simulink model "FLIGHT_Hexacopter_V2"  (R2025a)
settings: Solver=FixedStepDiscrete  StartTime=0.0  StopTime=inf  FixedStep=SampleTime_SAS  RelTol=1e-3  EnableMultiTasking=on
InitFcn:
  | Init_FLIGHT_Hexacopter
values from neighbouring files (symbols this model uses):
  d2r = pi/180    (= 0.0174532925199)    [Init_FLIGHT_Hexacopter.m]
  Kdrr = 0.004    [Init_FLIGHT_Hexacopter_fromNCMS.m]
  Kirr = 0.0    (= 0)    [Init_FLIGHT_Hexacopter_fromNCMS.m]
  Kpp = 3.3894    [Init_FLIGHT_Hexacopter_fromNCMS.m]
  Kpr = 3.3894    [Init_FLIGHT_Hexacopter_fromNCMS.m]
  Kprr = 0.1    [Init_FLIGHT_Hexacopter_fromNCMS.m]
  MAX_CONTROL_ANGLE_PITCH = 30*pi/180    (= 0.523598775598)    [Init_FLIGHT_Hexacopter.m]    (also in Init_FLIGHT_Hexacopter_fromNCMS.m = 0.349065850399)
  MAX_CONTROL_ANGLE_RATE_PITCH = 360*pi/180    (= 6.28318530718)    [Init_FLIGHT_Hexacopter.m]    (also in Init_FLIGHT_Hexacopter_fromNCMS.m)
  MAX_CONTROL_ANGLE_RATE_ROLL = 360*pi/180    (= 6.28318530718)    [Init_FLIGHT_Hexacopter.m]    (also in Init_FLIGHT_Hexacopter_fromNCMS.m)
  MAX_CONTROL_ANGLE_RATE_Y = 120*pi/180    (= 2.09439510239)    [Init_FLIGHT_Hexacopter.m]    (also in Init_FLIGHT_Hexacopter_fromNCMS.m)
  MAX_CONTROL_ANGLE_ROLL = 30*pi/180    (= 0.523598775598)    [Init_FLIGHT_Hexacopter.m]    (also in Init_FLIGHT_Hexacopter_fromNCMS.m = 0.349065850399)
  Nrr = 50    [Init_FLIGHT_Hexacopter_fromNCMS.m]
  PITCH_AUTHORITY = 1    [Init_FLIGHT_Hexacopter.m]
  ROLL_AUTHORITY = 1    [Init_FLIGHT_Hexacopter.m]
  SampleTime = 1/250    (= 0.004)    [Init_FLIGHT_Hexacopter.m]    (also in Init_FLIGHT_Hexacopter_fromNCMS.m = 0.01)
  SampleTime_SAS = 1/1000    (= 0.001)    [Init_FLIGHT_Hexacopter.m]
  YAW_AUTHORITY = 1    [Init_FLIGHT_Hexacopter.m]
undefined symbols (not defined in the file or in its folder): arguments, DiscIntNeverNeededParam, e_dot, event_sequence, fx, g1x, hx, id, integral_e, log_levels, MPC_Z_D, MPC_Z_I, MPC_Z_P, noutputs, omega, omega_dot, output, phi_cmd, phi_cmd_ddot, phi_cmd_dot, r, s, tau_roll, timestamp, w
libraries: px4Utilslib x65, simulink x21, px4uORBlib x12, slpidlib x9, cstblocks x5, simulink_extras x2, sharedtransform x1, px4Sensorslib x1, matrix_library x1, px4Peripheralslib x1
(part 1 of 3)
settings Model: ExtModeTrigDuration=10  Creator=sslee  LastModifiedBy=sslee
settings SolverCC: AlgebraicLoopSolver=TrustRegion  PositivePriorityOrder=on  MaxZcPerStep=1.0
settings OptimizationCC: EnhancedBackFolding=on  PassReuseOutputArgsAs=Individual arguments  ZeroExternalMemoryAtStartup=off  ZeroInternalMemoryAtStartup=off  MaxStackSize=64  OptimizeBlockOrder=speed  DifferentSizesBufferReuse=on  OptimizationCustomize=off  EfficientTunableParamExpr=on
settings DebuggingCC: ParameterTunabilityLossMsg=error  UnconnectedInputMsg=warning  UnconnectedOutputMsg=warning  UnconnectedLineMsg=warning  SymbolicDimsDataTypeCodeGenerationDiagnostic=none
settings HardwareCC: ProdBitPerPointer=32.0  ProdBitPerSizeT=32.0  ProdBitPerPtrDiffT=32.0  ProdLargestAtomicInteger=Long  ProdLargestAtomicFloat=Double  ProdWordSize=32.0  ProdLongLongMode=on  ProdHWDeviceType=ARM Compatible->ARM Cortex
settings ModelReferenceCC: EnableRefExpFcnMdlSchedulingChecks=on
settings SFSimCC: MATLABDynamicMemAlloc=off  SimTargetLang=C++  SimDLTargetLibrary=mkl-dnn
settings RTWCC: SystemTargetFile=ert.tlc  HardwareBoard=PX4 Pixhawk 6x  TLCOptions="-aInlineSetEventsForThisBaseRateFcn=TLC_FALSE -aSuppressMultiTaskScheduler=TLC_FALSE  -aRateBasedStepFcn=0"  TemplateMakefile=ert_default_tmf  GenerateReport=on  Toolchain=GNU Tools for PX4 Autopilots  IncludeHyperlinkInReport=on  LaunchReport=on  TargetLang=C++  GPUComputeCapability=3.5  DLArmComputeVersion=19.05  Description=Embedded Coder
settings CodeAppCC: ForceParamTrailComments=on  IgnoreCustomStorageClasses=off  OperatorAnnotations=on  SimulinkDataObjDesc=on  SFDataObjDesc=on  MATLABFcnDesc=on  InsertBlockDesc=on  BlockCommentType=BlockSIDComment  MATLABSourceComments=on
settings ERTTargetCC: ExtModeTransport=3.0  ExtModeStaticAllocSize=1024.0  InlinedParameterPlacement=Hierarchical  DynamicArrayContainerType=coder::array

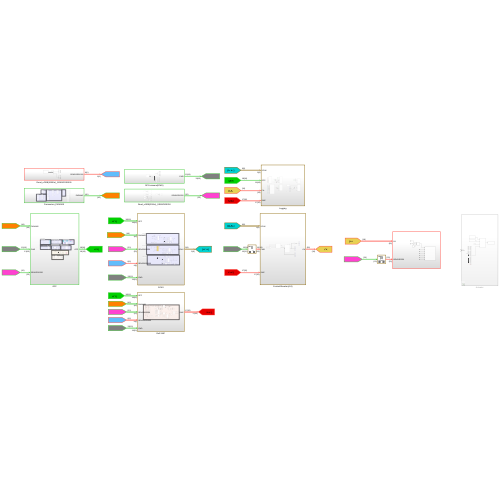
[thumbnail: Simulink's stored preview of the top-level diagram]
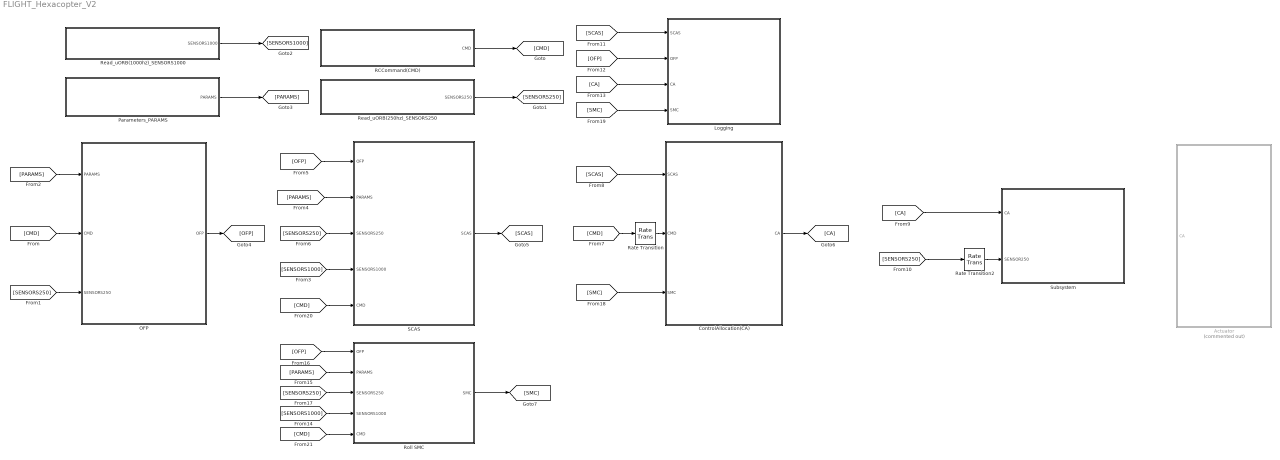
== system FLIGHT_Hexacopter_V2 ==
  Actuator : Subsystem  Commented=on
  ControlAllocation(CA) : Subsystem
  Logging : Subsystem
  OFP : Subsystem
  Parameters_PARAMS : Subsystem
  RCCommand(CMD) : Subsystem
  Rate Transition : RateTransition  OutPortSampleTime=SampleTime_SAS
  Rate Transition2 : RateTransition  OutPortSampleTime=SampleTime_SAS
  Read_uORB(1000hz)_SENSORS1000 : Subsystem
  Read_uORB(250hz)_SENSORS250 : Subsystem
  Roll SMC : Subsystem
  SCAS : Subsystem
  Subsystem : Subsystem
  wires:
  [SENSORS250] -> OFP/3(SENSORS250)
  Read_uORB(1000hz)_SENSORS1000/1(SENSORS1000) -> [SENSORS1000]
  RCCommand(CMD)/1(CMD) -> [CMD]
  Read_uORB(250hz)_SENSORS250/1(SENSORS250) -> [SENSORS250]
  [CMD] -> OFP/2(CMD)
  Parameters_PARAMS/1(PARAMS) -> [PARAMS]
  [PARAMS] -> OFP/1(PARAMS)
  OFP/1(OFP) -> [OFP]
  [OFP] -> SCAS/1(OFP)
  [PARAMS] -> SCAS/2(PARAMS)
  [SENSORS250] -> SCAS/3(SENSORS250)
  [SENSORS1000] -> SCAS/4(SENSORS1000)
  [CMD] -> Rate Transition/1
  SCAS/1(SCAS) -> [SCAS]
  [SCAS] -> ControlAllocation(CA)/1(SCAS)
  Rate Transition/1 -> ControlAllocation(CA)/2(CMD)
  ControlAllocation(CA)/1(CA) -> [CA]
  [SENSORS250] -> Rate Transition2/1
  [SCAS] -> Logging/1(SCAS)
  [OFP] -> Logging/2(OFP)
  [CA] -> Logging/3(CA)
  Rate Transition2/1 -> Subsystem/2(SENSOR250)
  [SENSORS250] -> Roll SMC/3(SENSORS250)
  [SENSORS1000] -> Roll SMC/4(SENSORS1000)
  [PARAMS] -> Roll SMC/2(PARAMS)
  [OFP] -> Roll SMC/1(OFP)
  Roll SMC/1(SMC) -> [SMC]
  [SMC] -> ControlAllocation(CA)/3(SMC)
  [SMC] -> Logging/4(SMC)
  [CMD] -> SCAS/5(CMD)
  [CMD] -> Roll SMC/5(CMD)
  [CA] -> Subsystem/1(CA)

== system FLIGHT_Hexacopter_V2/Actuator ==
  BusElementIn : Inport  PortName=CA  Element=thr_m1
  BusElementIn1 : Inport  PortName=CA  Element=thr_m2
  BusElementIn2 : Inport  PortName=CA  Element=thr_m3
  BusElementIn3 : Inport  PortName=CA  Element=thr_m4
  BusElementIn4 : Inport  PortName=CA  Element=thr_m5
  BusElementIn6 : Inport  PortName=CA  Element=thr_m6
  Bus Assignment : BusAssignment  AssignedSignals=timestamp,noutputs,output
  Constant : Constant  Value=6  OutDataTypeStr=uint32  SampleTime=SampleTime_SAS
  Ground : Ground
  Mux : Mux  Inputs=16
  PX4 Timestamp : px4Utilslib/PX4 Timestamp  SampleTime=0.01
  PX4 uORB Message : px4uORBlib/PX4 uORB Message  uORBTopic=ActuatorOutputs  SampleTime=SampleTime_SAS  selectInstance=actuator_outputs
  PX4 uORB Write : px4uORBlib/PX4 uORB Write  uORBTopic=ActuatorOutputs  selectInstance=actuator_outputs  MessageQueueLen=1
  wires:
  PX4 uORB Message/1 -> Bus Assignment/1
  Bus Assignment/1 -> PX4 uORB Write/1
  PX4 Timestamp/1 -> Bus Assignment/2
  Constant/1 -> Bus Assignment/3
  BusElementIn/1 -> Mux/1
  BusElementIn1/1 -> Mux/2
  BusElementIn2/1 -> Mux/3
  BusElementIn3/1 -> Mux/4
  BusElementIn4/1 -> Mux/5
  BusElementIn6/1 -> Mux/6
  Ground/1 -> Mux/15, Mux/14, Mux/13, Mux/12, Mux/11, Mux/10, Mux/9, Mux/8, Mux/7
  Mux/1 -> Bus Assignment/4

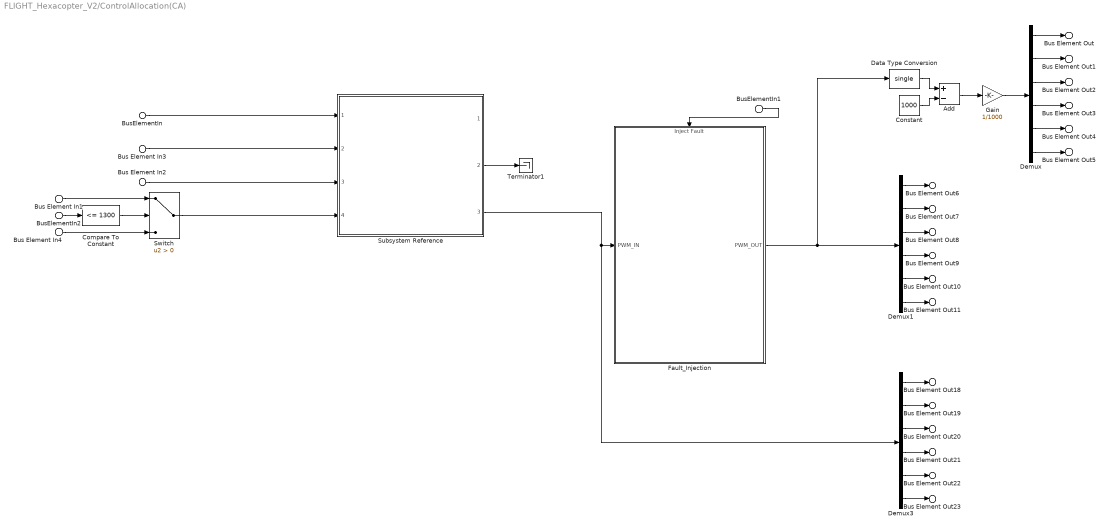
== system FLIGHT_Hexacopter_V2/ControlAllocation(CA) ==
  Bus Element In1 : Inport  PortName=SCAS  Element=tau_roll
  Bus Element In2 : Inport  PortName=SCAS  Element=tau_pitch
  Bus Element In3 : Inport  PortName=SCAS  Element=tau_yaw
  BusElementIn : Inport  PortName=SCAS  Element=tau_throttle
  BusElementIn1 : Inport  Port=2  PortName=CMD  Element=rc_inject_failure
  BusElementIn2 : Inport  Port=2  PortName=CMD  Element=rc_ctrl_switch
  Bus Element In4 : Inport  Port=3  PortName=SMC  Element=tau_roll
  Add : Sum  Inputs=+-
  Compare To Constant : simulink/Logic and Bit Operations/Compare To Constant  relop=<=  const=1300  OutDataTypeStr=boolean
  Constant : Constant  Value=1000  OutDataTypeStr=single  SampleTime=SampleTime_SAS
  Data Type Conversion : DataTypeConversion  OutDataTypeStr=single  SaturateOnIntegerOverflow=off  RndMeth=Floor
  Demux : Demux  Outputs=6
  Demux1 : Demux  Outputs=6
  Demux3 : Demux  Outputs=6
  Fault_Injection : Subsystem
      settings: PortSchema="{\"entries\":[{\"content\":{\"sides\":[{\"content\":{\"connectorIds\":[\"In1\"]},\"type\":\"ConnectorPlacement.EquallySpacedRectSide\",\"uuid\":\"fab26c65-8d77-46b7-b375-2033d08e8306\"},{\"content\":{\"connectorIds\":[\"Out1\"],\"side\":\"RIGHT\"},\"type\":\"ConnectorPlacement.EquallySpacedRectSide\",\"uuid\":\"bc3f50bd-e170-4b75-8089-4f92da68e83e\"},{\"content\":{\"connectorIds\":[\"In2\"],\"side\":\"TOP\"},\"type\":\"ConnectorPlacement.EquallySpacedRectSide\",\"uuid\":\"873ada90-6f93-48ab-a701-a52d28357753\"}]},\"type\":\"ConnectorPlacement.EquallySpacedConnector\",\"uuid\":\"201be8b3-bff4-4924-8e0c-28e5fee33d1c\"}],\"packageUris\":[\"http://schema.mathworks.com/mf0/Connector/R2020b\"],\"version\":\"1.0\"}"
  Gain : Gain  Gain=1/1000
  Subsystem Reference : Subsystem  ReferencedSubsystem=F550_ControlAllocation_sub_ver2023b
  Switch : Switch  Criteria=u2 > Threshold  SaturateOnIntegerOverflow=off  InputSameDT=off
  Terminator1 : Terminator
  Bus Element Out : Outport  PortName=CA  Element=thr_m1
  Bus Element Out1 : Outport  PortName=CA  Element=thr_m2
  Bus Element Out2 : Outport  PortName=CA  Element=thr_m3
  Bus Element Out3 : Outport  PortName=CA  Element=thr_m4
  Bus Element Out4 : Outport  PortName=CA  Element=thr_m5
  Bus Element Out5 : Outport  PortName=CA  Element=thr_m6
  Bus Element Out6 : Outport  PortName=CA  Element=pwm_after_fault_m1
  Bus Element Out7 : Outport  PortName=CA  Element=pwm_after_fault_m2
  Bus Element Out8 : Outport  PortName=CA  Element=pwm_after_fault_m3
  Bus Element Out9 : Outport  PortName=CA  Element=pwm_after_fault_m4
  Bus Element Out10 : Outport  PortName=CA  Element=pwm_after_fault_m5
  Bus Element Out11 : Outport  PortName=CA  Element=pwm_after_fault_m6
  Bus Element Out18 : Outport  PortName=CA  Element=pwm_before_fault_m1
  Bus Element Out19 : Outport  PortName=CA  Element=pwm_before_fault_m2
  Bus Element Out20 : Outport  PortName=CA  Element=pwm_before_fault_m3
  Bus Element Out21 : Outport  PortName=CA  Element=pwm_before_fault_m4
  Bus Element Out22 : Outport  PortName=CA  Element=pwm_before_fault_m5
  Bus Element Out23 : Outport  PortName=CA  Element=pwm_before_fault_m6
  wires:
  Demux/1 -> Bus Element Out/1
  Demux/2 -> Bus Element Out1/1
  Demux/3 -> Bus Element Out2/1
  Demux/4 -> Bus Element Out3/1
  Demux/5 -> Bus Element Out4/1
  Demux/6 -> Bus Element Out5/1
  Subsystem Reference/2 -> Terminator1/1
  BusElementIn1/1 -> Fault_Injection/2(Inject Fault)
  Fault_Injection/1(PWM_OUT) -> Data Type Conversion/1, Demux1/1
  Subsystem Reference/3 -> Demux3/1, Fault_Injection/1(PWM_IN)
  Demux1/1 -> Bus Element Out6/1
  Demux1/2 -> Bus Element Out7/1
  Demux1/3 -> Bus Element Out8/1
  Demux1/4 -> Bus Element Out9/1
  Demux1/5 -> Bus Element Out10/1
  Demux1/6 -> Bus Element Out11/1
  Demux3/1 -> Bus Element Out18/1
  Demux3/2 -> Bus Element Out19/1
  Demux3/3 -> Bus Element Out20/1
  Demux3/4 -> Bus Element Out21/1
  Demux3/5 -> Bus Element Out22/1
  Demux3/6 -> Bus Element Out23/1
  BusElementIn2/1 -> Compare To Constant/1
  Compare To Constant/1 -> Switch/2
  Bus Element In1/1 -> Switch/1
  Bus Element In4/1 -> Switch/3
  BusElementIn/1 -> Subsystem Reference/1
  Bus Element In3/1 -> Subsystem Reference/2
  Bus Element In2/1 -> Subsystem Reference/3
  Switch/1 -> Subsystem Reference/4
  Constant/1 -> Add/2
  Add/1 -> Gain/1
  Data Type Conversion/1 -> Add/1
  Gain/1 -> Demux/1

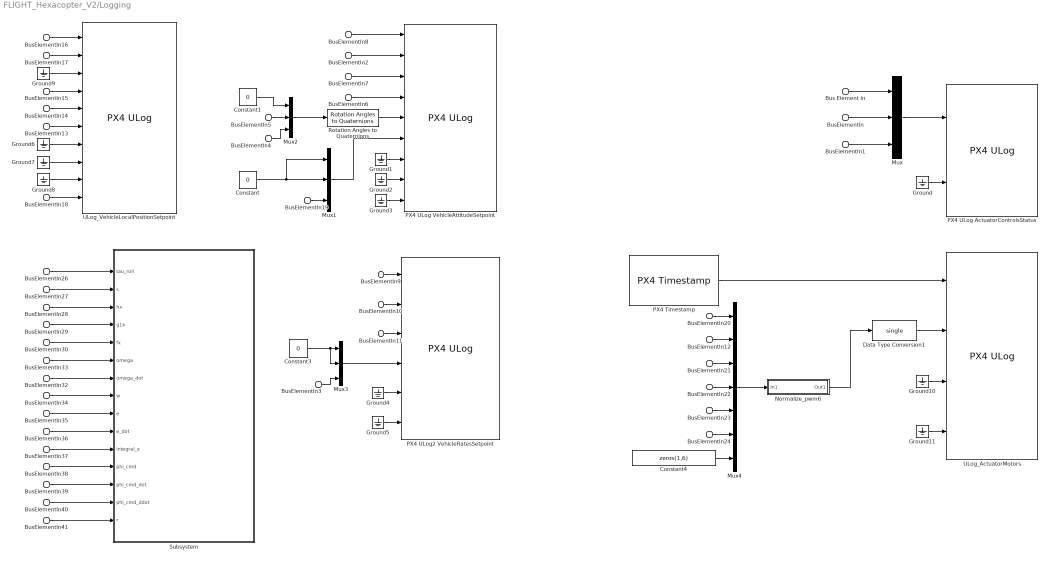
== system FLIGHT_Hexacopter_V2/Logging ==
  BusElementIn : Inport  PortName=SCAS  Element=tau_pitch
  BusElementIn1 : Inport  PortName=SCAS  Element=tau_yaw
  BusElementIn4 : Inport  PortName=SCAS  Element=des_roll
  BusElementIn8 : Inport  PortName=SCAS  Element=des_roll
  BusElementIn7 : Inport  PortName=SCAS  Element=des_roll
  BusElementIn5 : Inport  PortName=SCAS  Element=des_pitch
  BusElementIn2 : Inport  PortName=SCAS  Element=des_pitch
  BusElementIn6 : Inport  PortName=SCAS  Element=des_yr
  BusElementIn11 : Inport  PortName=SCAS  Element=des_yr
  BusElementIn9 : Inport  PortName=SCAS  Element=des_rollrate
  BusElementIn10 : Inport  PortName=SCAS  Element=des_pitchrate
  Bus Element In : Inport  PortName=SCAS  Element=tau_roll
  BusElementIn13 : Inport  Port=2  PortName=OFP  Element=ATL_des_vz
  BusElementIn14 : Inport  Port=2  PortName=OFP  Element=POS_des_vy
  BusElementIn15 : Inport  Port=2  PortName=OFP  Element=POS_des_vx
  BusElementIn16 : Inport  Port=2  PortName=OFP  Element=POS_des_x
  BusElementIn17 : Inport  Port=2  PortName=OFP  Element=POS_des_y
  BusElementIn18 : Inport  Port=2  PortName=OFP  Element=des_yr
  BusElementIn19 : Inport  Port=2  PortName=OFP  Element=des_thr
  BusElementIn3 : Inport  Port=2  PortName=OFP  Element=des_thr
  BusElementIn20 : Inport  Port=3  PortName=CA  Element=pwm_before_fault_m1
  BusElementIn12 : Inport  Port=3  PortName=CA  Element=pwm_before_fault_m2
  BusElementIn21 : Inport  Port=3  PortName=CA  Element=pwm_before_fault_m3
  BusElementIn22 : Inport  Port=3  PortName=CA  Element=pwm_before_fault_m4
  BusElementIn23 : Inport  Port=3  PortName=CA  Element=pwm_before_fault_m5
  BusElementIn24 : Inport  Port=3  PortName=CA  Element=pwm_before_fault_m6
  BusElementIn26 : Inport  Port=4  PortName=SMC  Element=tau_roll
  BusElementIn27 : Inport  Port=4  PortName=SMC  Element=s
  BusElementIn28 : Inport  Port=4  PortName=SMC  Element=hx
  BusElementIn29 : Inport  Port=4  PortName=SMC  Element=g1x_inv
  BusElementIn30 : Inport  Port=4  PortName=SMC  Element=fx
  BusElementIn32 : Inport  Port=4  PortName=SMC  Element=omega_phi_dot
  BusElementIn33 : Inport  Port=4  PortName=SMC  Element=omega_phi
  BusElementIn34 : Inport  Port=4  PortName=SMC  Element=w
  BusElementIn35 : Inport  Port=4  PortName=SMC  Element=e
  BusElementIn36 : Inport  Port=4  PortName=SMC  Element=e_dot
  BusElementIn37 : Inport  Port=4  PortName=SMC  Element=integral_e
  BusElementIn38 : Inport  Port=4  PortName=SMC  Element=phi_cmd
  BusElementIn39 : Inport  Port=4  PortName=SMC  Element=phi_cmd_dot
  BusElementIn40 : Inport  Port=4  PortName=SMC  Element=phi_cmd_ddot
  BusElementIn41 : Inport  Port=4  PortName=SMC  Element=r
  Constant : Constant  Value=0  OutDataTypeStr=single  SampleTime=SampleTime
  Constant1 : Constant  Value=0  OutDataTypeStr=single  SampleTime=SampleTime
  Constant3 : Constant  Value=0  OutDataTypeStr=single
  Constant4 : Constant  Value=zeros(1,6)  OutDataTypeStr=uint16  SampleTime=SampleTime_SAS
  Data Type Conversion1 : DataTypeConversion  OutDataTypeStr=single  SaturateOnIntegerOverflow=off  RndMeth=Floor
  Ground{,1..11} (12 alike) : Ground
  Mux{,1..3} (4 alike) : Mux  Inputs=3
  Mux4 : Mux  Inputs=7
  Normalize_pwm6 : Subsystem
  PX4 Timestamp : px4Utilslib/PX4 Timestamp  SampleTime=SampleTime_SAS
  PX4 ULog ActuatorControlsStatus : px4Utilslib/PX4 ULog  uORBTopic=ActuatorControlsStatus
  PX4 ULog VehicleAttitudeSetpoint : px4Utilslib/PX4 ULog  uORBTopic=VehicleAttitudeSetpoint
  PX4 ULog2 VehicleRatesSetpoint : px4Utilslib/PX4 ULog  uORBTopic=VehicleRatesSetpoint
  Rotation Angles to Quaternions : sharedtransform/Rotation Angles to Quaternions  rotationOrder=ZYX  aMode=aMode
  Subsystem : Subsystem
  ULog_ActuatorMotors : px4Utilslib/PX4 ULog  uORBTopic=ActuatorMotors
  ULog_VehicleLocalPositionSetpoint : px4Utilslib/PX4 ULog  uORBTopic=VehicleLocalPositionSetpoint
  wires:
  BusElementIn1/1 -> Mux/3
  Bus Element In/1 -> Mux/1
  BusElementIn/1 -> Mux/2
  BusElementIn4/1 -> Mux2/3
  Constant1/1 -> Mux2/1
  Mux2/1 -> Rotation Angles to Quaternions/1
  BusElementIn5/1 -> Mux2/2
  Constant/1 -> Mux1/1, Mux1/2
  BusElementIn19/1 -> Mux1/3
  BusElementIn3/1 -> Mux3/3
  Constant3/1 -> Mux3/2, Mux3/1
  BusElementIn20/1 -> Mux4/1
  BusElementIn21/1 -> Mux4/3
  BusElementIn22/1 -> Mux4/4
  Normalize_pwm6/1(Out1) -> Data Type Conversion1/1
  Constant4/1 -> Mux4/7
  BusElementIn12/1 -> Mux4/2
  BusElementIn23/1 -> Mux4/5
  BusElementIn24/1 -> Mux4/6
  Mux4/1 -> Normalize_pwm6/1(In1)
  Data Type Conversion1/1 -> ULog_ActuatorMotors/2
  PX4 Timestamp/1 -> ULog_ActuatorMotors/1
  Ground10/1 -> ULog_ActuatorMotors/3
  Ground11/1 -> ULog_ActuatorMotors/4
  Mux/1 -> PX4 ULog ActuatorControlsStatus/1
  Ground/1 -> PX4 ULog ActuatorControlsStatus/2
  BusElementIn8/1 -> PX4 ULog VehicleAttitudeSetpoint/1
  BusElementIn6/1 -> PX4 ULog VehicleAttitudeSetpoint/4
  Rotation Angles to Quaternions/1 -> PX4 ULog VehicleAttitudeSetpoint/5
  Ground1/1 -> PX4 ULog VehicleAttitudeSetpoint/7
  Ground2/1 -> PX4 ULog VehicleAttitudeSetpoint/8
  Mux1/1 -> PX4 ULog VehicleAttitudeSetpoint/6
  BusElementIn16/1 -> ULog_VehicleLocalPositionSetpoint/1
  BusElementIn17/1 -> ULog_VehicleLocalPositionSetpoint/2
  BusElementIn15/1 -> ULog_VehicleLocalPositionSetpoint/4
  BusElementIn14/1 -> ULog_VehicleLocalPositionSetpoint/5
  BusElementIn13/1 -> ULog_VehicleLocalPositionSetpoint/6
  Ground6/1 -> ULog_VehicleLocalPositionSetpoint/7
  Ground7/1 -> ULog_VehicleLocalPositionSetpoint/8
  Ground8/1 -> ULog_VehicleLocalPositionSetpoint/9
  BusElementIn18/1 -> ULog_VehicleLocalPositionSetpoint/10
  BusElementIn10/1 -> PX4 ULog2 VehicleRatesSetpoint/2
  BusElementIn11/1 -> PX4 ULog2 VehicleRatesSetpoint/3
  BusElementIn9/1 -> PX4 ULog2 VehicleRatesSetpoint/1
  Mux3/1 -> PX4 ULog2 VehicleRatesSetpoint/4
  Ground4/1 -> PX4 ULog2 VehicleRatesSetpoint/5
  Ground5/1 -> PX4 ULog2 VehicleRatesSetpoint/6
  Ground9/1 -> ULog_VehicleLocalPositionSetpoint/3
  BusElementIn2/1 -> PX4 ULog VehicleAttitudeSetpoint/2
  BusElementIn7/1 -> PX4 ULog VehicleAttitudeSetpoint/3
  Ground3/1 -> PX4 ULog VehicleAttitudeSetpoint/9
  BusElementIn27/1 -> Subsystem/2(s)
  BusElementIn28/1 -> Subsystem/3(hx)
  BusElementIn29/1 -> Subsystem/4(g1x)
  BusElementIn30/1 -> Subsystem/5(fx)
  BusElementIn34/1 -> Subsystem/8(w)
  BusElementIn35/1 -> Subsystem/9(e)
  BusElementIn36/1 -> Subsystem/10(e_dot)
  BusElementIn37/1 -> Subsystem/11(integral_e)
  BusElementIn38/1 -> Subsystem/12(phi_cmd)
  BusElementIn39/1 -> Subsystem/13(phi_cmd_dot)
  BusElementIn40/1 -> Subsystem/14(phi_cmd_ddot)
  BusElementIn41/1 -> Subsystem/15(r)
  BusElementIn26/1 -> Subsystem/1(tau_roll)
  BusElementIn33/1 -> Subsystem/6(omega)
  BusElementIn32/1 -> Subsystem/7(omega_dot)

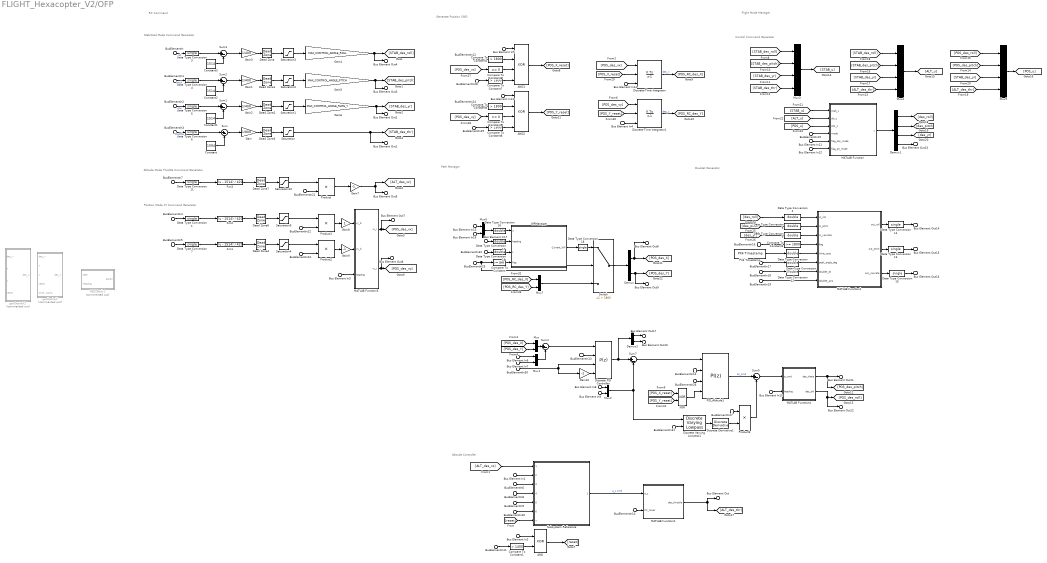
== system FLIGHT_Hexacopter_V2/OFP ==
  note: Doublet Generator
  note: Control Command Generator
  note: Altitude Controller
  note: Position Mode XY Command Generator
  note: Altitude Mode Throttle Command Generator
  note: Stabilized Mode Command Generator
  note: RC Command
  note: Flight Mode Manager
  note: Generate Position CMD
  note: Path Manager
  BusElementIn6 : Inport  PortName=PARAMS  Element=MPC_Z_VEL_P_ACC
  BusElementIn8 : Inport  PortName=PARAMS  Element=MPC_Z_VEL_I_ACC
  BusElementIn9 : Inport  PortName=PARAMS  Element=MPC_Z_VEL_D_ACC
  BusElementIn10 : Inport  PortName=PARAMS  Element=MPC_THR_HOVER
  BusElementIn14 : Inport  PortName=PARAMS  Element=MPC_XY_VEL_P_ACC
  BusElementIn17 : Inport  PortName=PARAMS  Element=DOUBLET_PEAK_ANG
  BusElementIn18 : Inport  PortName=PARAMS  Element=DOUBLET_DT
  BusElementIn19 : Inport  PortName=PARAMS  Element=DOUBLET_AXIS
  BusElementIn20 : Inport  PortName=PARAMS  Element=IMU_DGYRO_CUTOFF
  BusElementIn31 : Inport  PortName=PARAMS  Element=IMU_DGYRO_CUTOFF
  BusElementIn21 : Inport  PortName=PARAMS  Element=MPC_Z_VEL_MAX_UP
  BusElementIn22 : Inport  PortName=PARAMS  Element=MPC_XY_VEL_MAX
  BusElementIn23 : Inport  PortName=PARAMS  Element=MPC_XY_VEL_MAX
  BusElementIn30 : Inport  PortName=PARAMS  Element=MPC_XY_VEL_MAX
  BusElementIn26 : Inport  PortName=PARAMS  Element=MPC_XY_VEL_I_ACC
  BusElementIn27 : Inport  PortName=PARAMS  Element=MPC_XY_VEL_D_ACC
  BusElementIn13 : Inport  PortName=PARAMS  Element=MPC_XY_P
  BusElementIn32 : Inport  PortName=PARAMS  Element=MPC_WP_LENGTH
  BusElementIn2 : Inport  Port=2  PortName=CMD  Element=rc_mode2_yaw
  BusElementIn{11..12,15,24} (4 alike) : Inport  Port=2  PortName=CMD  Element=rc_mode
  BusElementIn16 : Inport  Port=2  PortName=CMD  Element=rc_doublet
  BusElementIn25 : Inport  Port=2  PortName=CMD  Element=rc_ap_sw
  BusElementIn28 : Inport  Port=2  PortName=CMD  Element=rc_ap_sw
  BusElementIn29 : Inport  Port=2  PortName=CMD  Element=rc_ap_sw
  BusElementIn : Inport  Port=2  PortName=CMD  Element=rc_mode2_roll
  BusElementIn4 : Inport  Port=2  PortName=CMD  Element=rc_mode2_roll
  BusElementIn1 : Inport  Port=2  PortName=CMD  Element=rc_mode2_pitch
  BusElementIn5 : Inport  Port=2  PortName=CMD  Element=rc_mode2_pitch
  BusElementIn3 : Inport  Port=2  PortName=CMD  Element=rc_mode2_throttle
  BusElementIn7 : Inport  Port=2  PortName=CMD  Element=rc_mode2_throttle
  Bus Element In1 : Inport  Port=3  PortName=SENSORS250  Element=W
  Bus Element In2 : Inport  Port=3  PortName=SENSORS250  Element=VehicleStatus_armed
  Bus Element In5 : Inport  Port=3  PortName=SENSORS250  Element=VehicleStatus_armed
  Bus Element In13 : Inport  Port=3  PortName=SENSORS250  Element=VehicleStatus_armed
  Bus Element In14 : Inport  Port=3  PortName=SENSORS250  Element=X
  Bus Element In6 : Inport  Port=3  PortName=SENSORS250  Element=X
  Bus Element In15 : Inport  Port=3  PortName=SENSORS250  Element=X
  Bus Element In4 : Inport  Port=3  PortName=SENSORS250  Element=Y
  Bus Element In7 : Inport  Port=3  PortName=SENSORS250  Element=Y
  Bus Element In16 : Inport  Port=3  PortName=SENSORS250  Element=Y
  Bus Element In8 : Inport  Port=3  PortName=SENSORS250  Element=U
  Bus Element In9 : Inport  Port=3  PortName=SENSORS250  Element=V
  Bus Element In10 : Inport  Port=3  PortName=SENSORS250  Element=Heading
  Bus Element In3 : Inport  Port=3  PortName=SENSORS250  Element=Heading
  Bus Element In17 : Inport  Port=3  PortName=SENSORS250  Element=Heading
  Bus Element In11 : Inport  Port=3  PortName=SENSORS250  Element=VehicleStatus_flag_position_mode
  Bus Element In12 : Inport  Port=3  PortName=SENSORS250  Element=VehicleStatus_flag_altitude_mode
  AND : Logic  Operator=XOR  AllPortsSameDT=off  OutDataTypeStr=boolean
  AND1 : Logic  Operator=XOR  Inputs=4  AllPortsSameDT=off  OutDataTypeStr=boolean
  AND2 : Logic  Operator=XOR  Inputs=4  AllPortsSameDT=off  OutDataTypeStr=boolean
  Compare To Constant : simulink/Logic and Bit Operations/Compare To Constant  relop=>=  const=1800  OutDataTypeStr=boolean
  Compare To Constant1 : simulink/Logic and Bit Operations/Compare To Constant  relop=>  const=1400  OutDataTypeStr=boolean
  Compare To Constant{2,4,7..8} (4 alike) : simulink/Logic and Bit Operations/Compare To Constant  relop=>  const=1800  OutDataTypeStr=boolean
  Compare To Constant3 : simulink/Logic and Bit Operations/Compare To Constant  relop=>=  const=1800  OutDataTypeStr=boolean
  Compare To Constant5 : simulink/Logic and Bit Operations/Compare To Constant  relop===  const=0  OutDataTypeStr=boolean
  Compare To Constant6 : simulink/Logic and Bit Operations/Compare To Constant  relop===  const=0  OutDataTypeStr=boolean
  Constant : Constant  Value=1094
  Constant1 : Constant  Value=1514  OutDataTypeStr=single
  Constant2 : Constant  Value=1514  OutDataTypeStr=single
  Constant3 : Constant  Value=1514  OutDataTypeStr=single
  Data Type Conversion{,2,8..10,12,16..17,19} (9 alike) : DataTypeConversion  OutDataTypeStr=double  SaturateOnIntegerOverflow=off  RndMeth=Floor
  Data Type Conversion{1,3..7,11,13..15,18} (11 alike) : DataTypeConversion  OutDataTypeStr=single  SaturateOnIntegerOverflow=off  RndMeth=Floor
  Dead Zone{,1..3} (4 alike) : DeadZone  LowerValue=-0.005  UpperValue=0.005
  Dead Zone4 : DeadZone  LowerValue=-0.05  UpperValue=0.05
  Dead Zone6 : DeadZone  LowerValue=-0.05  UpperValue=0.05
  Dead Zone7 : DeadZone  LowerValue=-0.1  UpperValue=0.1
  Demux : Demux  Outputs=2
  Demux1 : Demux
  Demux2 : Demux  Outputs=2
  Discrete Derivative1 : simulink/Discrete/Discrete Derivative  gainval=1.0  ICPrevScaledInput=0.0  OutMin=[]  OutMax=[]  OutDataType=fixdt(1, 16)  OutScaling=2^-10  DoSatur=off
  Discrete PID Controller : slpidlib/PID Controller  Controller=P  Form=Parallel  TimeDomain=Discrete-time  UseExternalTs=off  SampleTime=SampleTime  IntegratorMethod=Forward Euler  FilterMethod=Forward Euler  ControllerParametersSource=external  P=1  I=1  UseKiTs=off  D=0  UseExternalDerivativeSource=off  N=100  UseFilter=on  TunerSelectOption=Transfer Function Based (PID Tuner App)  InitialConditionSource=internal  InitialConditionForIntegrator=0  InitialConditionForFilter=0  DifferentiatorICPrevScaledInput=0  ExternalReset=none  TrackingMode=off  Kt=1  LimitOutput=on  SatLimitsSource=external  UpperSaturationLimit=5  LowerSaturationLimit=-5  LinearizeAsGain=off  AntiWindupMode=none  Kb=1  LimitIntegrator=off  UpperIntegratorSaturationLimit=inf  LowerIntegratorSaturationLimit=-inf  POutMin=[]  POutMax=[]  IOutMin=[]  IOutMax=[]  DOutMin=[]  DOutMax=[]  NOutMin=[]  NOutMax=[]  SumOutMin=[]  SumOutMax=[]  SaturationOutMin=[]  SaturationOutMax=[]  PParamMin=[]  PParamMax=[]  IParamMin=[]  IParamMax=[]  DParamMin=[]  DParamMax=[]  NParamMin=[]  NParamMax=[]  KbParamMin=[]  KbParamMax=[]  KtParamMin=[]  KtParamMax=[]  KbOutMin=[]  KbOutMax=[]  KtOutMin=[]  KtOutMax=[]  IntegratorOutMin=[]  IntegratorOutMax=[]  FilterOutMin=[]  FilterOutMax=[]  SumI1OutMin=[]  SumI1OutMax=[]  SumI2OutMin=[]  SumI2OutMax=[]  SumI3OutMin=[]  SumI3OutMax=[]  SumI4OutMin=[]  SumI4OutMax=[]  SumDOutMin=[]  SumDOutMax=[]  DifferentiatorOutMin=[]  DifferentiatorOutMax=[]  FilterDiffOutCoefMin=[]  FilterDiffOutCoefMax=[]  ReciprocalOutMin=[]  ReciprocalOutMax=[]  SumDenOutMin=[]  SumDenOutMax=[]  SumNumOutMin=[]  SumNumOutMax=[]  DivideOutMin=[]  DivideOutMax=[]  UdiffTsProdOutMin=[]  UdiffTsProdOutMax=[]  NTsProdOutMin=[]  NTsProdOutMax=[]  UintegralTsProdOutMin=[]  UintegralTsProdOutMax=[]  UngainTsProdOutMin=[]  UngainTsProdOutMax=[]  ClampingZeroOutDataTypeStr=Inherit: Inherit via back propagation  ClampingZeroOutMin=[]  ClampingZeroOutMax=[]  FilterDenConstantOutDataTypeStr=Inherit: Inherit via back propagation  FilterDenConstantOutMin=[]  FilterDenConstantOutMax=[]  PCopyOutDataTypeStr=Inherit: Inherit via back propagation  PCopyOutMin=[]  PCopyOutMax=[]  NCopyOutDataTypeStr=Inherit: Inherit via back propagation  NCopyOutMin=[]  NCopyOutMax=[]  IntegratorContinuousStateAttributes=''  IntegratorStateMustResolveToSignalObject=off  IntegratorRTWStateStorageClass=Auto  FilterContinuousStateAttributes=''  FilterStateMustResolveToSignalObject=off  FilterRTWStateStorageClass=Auto  ParallelPVariant=ExternalParameters  IdealPVariant=Disabled  IVariant=Disabled  DVariant=Disabled  IntegratorVariant=Disabled  SatVariant=External  AWVariant=Disabled  PCopyVariant=Disabled  TRVariant=Disabled  FdbkBlocksVariant=Forward  IdealPFdbkVariant=Disabled  SatFdbkVariant=Disabled  DerivativeFilterVariant=Disabled  NVariant=Disabled  NCopyVariant=Disabled_SignalSpec  FilterICVariant=Disabled  IntegratorICVariant=Disabled  ExternalResetVariant=Disabled  TRSumVariant=Passthrough  SumFdbkVariant=Disabled  SumVariant=Passthrough_P  TsampFilterVariant=InternalTs  TsampNgainVariant=Passthrough  TsampIntegralVariant=Disabled_SignalSpec  ExternalSaturationOutDataTypeStr=Inherit: Same as second input  DerivativeSourceVariant=Disabled  PreIntVariant=InternalPreInt
      settings: LibrarySourceBlock=simulink/Discrete/Discrete PID Controller
  Discrete Varying Lowpass1 : cstblocks/Linear Parameter Varying/Discrete Varying Lowpass  N=2  w0=0  Ts=SampleTime
  Discrete-Time Integrator : DiscreteIntegrator  ExternalReset=either  InitialConditionSource=external  InitialCondition=SampleTime  SampleTime=SampleTime  UpperSaturationLimit=+10  LowerSaturationLimit=-50  ICPrevOutput=DiscIntNeverNeededParam  ICPrevScaledInput=DiscIntNeverNeededParam
  Discrete-Time Integrator1 : DiscreteIntegrator  ExternalReset=either  InitialConditionSource=external  InitialCondition=SampleTime  SampleTime=SampleTime  UpperSaturationLimit=+10  LowerSaturationLimit=-50  ICPrevOutput=DiscIntNeverNeededParam  ICPrevScaledInput=DiscIntNeverNeededParam
  Fcn1 : Fcn  Expr=(u - 1514) / 420
  Fcn2 : Fcn  Expr=(u - 1514) / 420
  Fcn3 : Fcn  Expr=(u - 1514) / 420
  Gain : Gain  Gain=1/800  OutDataTypeStr=single
  Gain1 : Gain  Gain=1/400  OutDataTypeStr=single
  Gain10 : Gain  Gain=-1
  Gain2 : Gain  Gain=1/400  OutDataTypeStr=single
  Gain3 : Gain  Gain=1/400  OutDataTypeStr=single
  Gain4 : Gain  Gain=MAX_CONTROL_ANGLE_ROLL
  Gain5 : Gain  Gain=MAX_CONTROL_ANGLE_PITCH
  Gain6 : Gain  Gain=MAX_CONTROL_ANGLE_RATE_Y
  Gain7 : Gain  Gain=-1
  Gain8 : Gain
  Gain9 : Gain  Gain=-1
  MATLAB Function : MATLAB Function  TreatAsAtomicUnit=on
  MATLAB Function1 : MATLAB Function  TreatAsAtomicUnit=on
  MATLAB Function2 : MATLAB Function  TreatAsAtomicUnit=on
  MATLAB Function3 : MATLAB Function  TreatAsAtomicUnit=on
  MATLAB Function4 : MATLAB Function  TreatAsAtomicUnit=on
  Mux{,1..2,6..7} (5 alike) : Mux  Inputs=2
  Mux3 : Mux
  Mux4 : Mux
  Mux5 : Mux
  NED2Body1 : Subsystem  Commented=on
  PID_Altitude1 : slpidlib/PID Controller  Controller=PI  Form=Parallel  TimeDomain=Discrete-time  UseExternalTs=off  SampleTime=SampleTime  IntegratorMethod=Backward Euler  FilterMethod=Forward Euler  ControllerParametersSource=external  P=MPC_Z_P  I=MPC_Z_I  UseKiTs=off  D=MPC_Z_D  UseExternalDerivativeSource=off  N=10  UseFilter=on  TunerSelectOption=Transfer Function Based (PID Tuner App)  InitialConditionSource=internal  InitialConditionForIntegrator=0  InitialConditionForFilter=0  DifferentiatorICPrevScaledInput=0  ExternalReset=either  TrackingMode=off  Kt=1  LimitOutput=off  SatLimitsSource=internal  UpperSaturationLimit=30*d2r  LowerSaturationLimit=-30*d2r  LinearizeAsGain=off  AntiWindupMode=clamping  Kb=1  LimitIntegrator=on  UpperIntegratorSaturationLimit=30*d2r*0.3  LowerIntegratorSaturationLimit=-30*d2r*0.3  POutMin=[]  POutMax=[]  IOutMin=[]  IOutMax=[]  DOutMin=[]  DOutMax=[]  NOutMin=[]  NOutMax=[]  SumOutMin=[]  SumOutMax=[]  SaturationOutMin=[]  SaturationOutMax=[]  PParamMin=[]  PParamMax=[]  IParamMin=[]  IParamMax=[]  DParamMin=[]  DParamMax=[]  NParamMin=[]  NParamMax=[]  KbParamMin=[]  KbParamMax=[]  KtParamMin=[]  KtParamMax=[]  KbOutMin=[]  KbOutMax=[]  KtOutMin=[]  KtOutMax=[]  IntegratorOutMin=[]  IntegratorOutMax=[]  FilterOutMin=[]  FilterOutMax=[]  SumI1OutMin=[]  SumI1OutMax=[]  SumI2OutMin=[]  SumI2OutMax=[]  SumI3OutMin=[]  SumI3OutMax=[]  SumI4OutMin=[]  SumI4OutMax=[]  SumDOutMin=[]  SumDOutMax=[]  DifferentiatorOutMin=[]  DifferentiatorOutMax=[]  FilterDiffOutCoefMin=[]  FilterDiffOutCoefMax=[]  ReciprocalOutMin=[]  ReciprocalOutMax=[]  SumDenOutMin=[]  SumDenOutMax=[]  SumNumOutMin=[]  SumNumOutMax=[]  DivideOutMin=[]  DivideOutMax=[]  UdiffTsProdOutMin=[]  UdiffTsProdOutMax=[]  NTsProdOutMin=[]  NTsProdOutMax=[]  UintegralTsProdOutMin=[]  UintegralTsProdOutMax=[]  UngainTsProdOutMin=[]  UngainTsProdOutMax=[]  ClampingZeroOutDataTypeStr=Inherit: Inherit via back propagation  ClampingZeroOutMin=[]  ClampingZeroOutMax=[]  FilterDenConstantOutDataTypeStr=Inherit: Inherit via back propagation  FilterDenConstantOutMin=[]  FilterDenConstantOutMax=[]  PCopyOutDataTypeStr=Inherit: Inherit via back propagation  PCopyOutMin=[]  PCopyOutMax=[]  NCopyOutDataTypeStr=Inherit: Inherit via back propagation  NCopyOutMin=[]  NCopyOutMax=[]  IntegratorContinuousStateAttributes=''  IntegratorStateMustResolveToSignalObject=off  IntegratorRTWStateStorageClass=Auto  FilterContinuousStateAttributes=''  FilterStateMustResolveToSignalObject=off  FilterRTWStateStorageClass=Auto  ParallelPVariant=ExternalParameters  IdealPVariant=Disabled  IVariant=ExternalParameters  DVariant=Disabled  IntegratorVariant=Discrete  SatVariant=Disabled  AWVariant=Passthrough  PCopyVariant=Disabled  TRVariant=Disabled  FdbkBlocksVariant=Forward  IdealPFdbkVariant=Disabled  SatFdbkVariant=Disabled  DerivativeFilterVariant=Disabled  NVariant=Disabled  NCopyVariant=Disabled_SignalSpec  FilterICVariant=Disabled  IntegratorICVariant=InternalICs  ExternalResetVariant=ExternalReset  TRSumVariant=Passthrough  SumFdbkVariant=Disabled  SumVariant=Sum_PI  TsampFilterVariant=InternalTs  TsampNgainVariant=Passthrough  TsampIntegralVariant=Disabled_SignalSpec  ExternalSaturationOutDataTypeStr=Inherit: Same as second input  DerivativeSourceVariant=Disabled  PreIntVariant=InternalPreInt
  PX4 Timestamp : px4Utilslib/PX4 Timestamp  SampleTime=SampleTime
  Product{,1..3} (4 alike) : Product
  Saturation : Saturate  UpperLimit=0.90  LowerLimit=0
  Saturation{1..4,9..10} (6 alike) : Saturate  UpperLimit=1  LowerLimit=-1
  Subsystem Reference : Subsystem  ReferencedSubsystem=CAS_PI_slash_D_Controller
  Sum{,1..5,7} (7 alike) : Sum  Inputs=|+-
  Switch : Switch  Criteria=u2 > Threshold  Threshold=1800  SaturateOnIntegerOverflow=off  InputSameDT=off
  WPManager : MATLAB Function  TreatAsAtomicUnit=on
  XOR : Logic  Operator=XOR  AllPortsSameDT=off  OutDataTypeStr=boolean
  genDesireX : MATLAB Function  Commented=on  TreatAsAtomicUnit=on
  genDesireX1 : MATLAB Function  Commented=on  TreatAsAtomicUnit=on
  Bus Element Out : Outport  PortName=OFP  Element=ALT_des_thr
  Bus Element Out1 : Outport  PortName=OFP  Element=STAB_des_thr
  Bus Element Out2 : Outport  PortName=OFP  Element=STAB_des_yr
  Bus Element Out3 : Outport  PortName=OFP  Element=STAB_des_pitch
  Bus Element Out4 : Outport  PortName=OFP  Element=STAB_des_roll
  Bus Element Out5 : Outport  PortName=OFP  Element=ATL_des_vz
  Bus Element Out6 : Outport  PortName=OFP  Element=POS_des_vy
  Bus Element Out7 : Outport  PortName=OFP  Element=POS_des_vx
  Bus Element Out8 : Outport  PortName=OFP  Element=POS_des_x
  Bus Element Out9 : Outport  PortName=OFP  Element=POS_des_y
  Bus Element Out10 : Outport  PortName=OFP  Element=POS_des_V
  Bus Element Out11 : Outport  PortName=OFP  Element=POS_des_pitch
  Bus Element Out12 : Outport  PortName=OFP  Element=POS_des_roll
  Bus Element Out13 : Outport  PortName=OFP  Element=des_thr
  Bus Element Out14 : Outport  PortName=OFP  Element=des_roll
  Bus Element Out15 : Outport  PortName=OFP  Element=des_pitch
  Bus Element Out16 : Outport  PortName=OFP  Element=des_yr
  Bus Element Out17 : Outport  PortName=OFP  Element=POS_des_U
  wires:
  Gain6/1 -> Bus Element Out2/1, [STAB_des_yr]
  Gain/1 -> Dead Zone3/1
  Sum2/1 -> Gain1/1
  BusElementIn3/1 -> Data Type Conversion6/1  "throttle"
  Saturation1/1 -> Gain6/1
  BusElementIn2/1 -> Data Type Conversion5/1  "yaw"
  Dead Zone/1 -> Saturation3/1
  Constant/1 -> Sum/2
  Constant3/1 -> Sum3/2
  BusElementIn/1 -> Data Type Conversion3/1  "roll"
  Constant2/1 -> Sum2/2
  Sum1/1 -> Gain2/1
  Sum/1 -> Gain/1
  Sum3/1 -> Gain3/1
  Dead Zone1/1 -> Saturation2/1
  BusElementIn1/1 -> Data Type Conversion4/1  "pitch"
  Dead Zone2/1 -> Saturation1/1
  Saturation2/1 -> Gain5/1
  Constant1/1 -> Sum1/2
  Gain1/1 -> Dead Zone1/1
  Gain2/1 -> Dead Zone2/1
  Dead Zone3/1 -> Saturation/1
  Saturation3/1 -> Gain4/1
  Gain3/1 -> Dead Zone/1
  Saturation/1 -> Bus Element Out1/1, [STAB_des_thr]
  Gain5/1 -> Bus Element Out3/1, [STAB_des_pitch]
  Gain4/1 -> Bus Element Out4/1, [STAB_des_roll]
  Dead Zone7/1 -> Saturation10/1
  Fcn3/1 -> Dead Zone7/1
  Data Type Conversion11/1 -> Fcn3/1
  Saturation10/1 -> Product/1
  Product/1 -> Gain7/1
  BusElementIn7/1 -> Data Type Conversion11/1
  Data Type Conversion3/1 -> Sum3/1
  Data Type Conversion4/1 -> Sum2/1
  Data Type Conversion5/1 -> Sum1/1
  Data Type Conversion6/1 -> Sum/1
  Data Type Conversion7/1 -> Fcn1/1
  Fcn2/1 -> Dead Zone6/1
  Product2/1 -> Gain9/1
  BusElementIn5/1 -> Data Type Conversion7/1
  Saturation9/1 -> Product1/1
  Saturation4/1 -> Product2/1
  Dead Zone6/1 -> Saturation9/1
  Data Type Conversion1/1 -> Fcn2/1
  Dead Zone4/1 -> Saturation4/1
  Fcn1/1 -> Dead Zone4/1
  BusElementIn4/1 -> Data Type Conversion1/1
  Product1/1 -> Gain8/1
  BusElementIn11/1 -> Compare To Constant1/1
  Compare To Constant1/1 -> AND/2
  AND/1 -> [reset]
  Bus Element In2/1 -> AND/1
  Discrete-Time Integrator/1 -> [POS_RC_des_X]  "des_x"
  [POS_X_reset] -> Discrete-Time Integrator/2
  [POS_des_vx] -> Discrete-Time Integrator/1
  [POS_des_vy] -> Discrete-Time Integrator1/1
  [POS_Y_reset] -> Discrete-Time Integrator1/2
  Compare To Constant2/1 -> AND1/2
  AND1/1 -> [POS_X_reset]
  BusElementIn12/1 -> Compare To Constant2/1
  Bus Element In5/1 -> AND1/1
  Bus Element In8/1 -> Mux2/1
  Bus Element In9/1 -> Mux2/2
  Mux2/1 -> Sum7/2, Discrete Varying Lowpass1/1
  BusElementIn14/1 -> PID_Altitude1/2
  [STAB_des_roll] -> Mux3/1
  [STAB_des_pitch] -> Mux3/2
  [STAB_des_yr] -> Mux3/3
  [STAB_des_thr] -> Mux3/4
  Mux3/1 -> [STAB_u]
  [STAB_des_roll] -> Mux4/1
  [STAB_des_pitch] -> Mux4/2
  [STAB_des_yr] -> Mux4/3
  [ALT_des_thr] -> Mux4/4
  Mux4/1 -> [ALT_u]
  Mux5/1 -> [POS_u]
  [POS_des_roll] -> Mux5/1
  [POS_des_pitch] -> Mux5/2
  [STAB_des_yr] -> Mux5/3
  [ALT_des_thr] -> Mux5/4
  [STAB_u] -> MATLAB Function/1(stab_u)
  [ALT_u] -> MATLAB Function/2(alt_u)
  [POS_u] -> MATLAB Function/3(pos_u)
  BusElementIn15/1 -> MATLAB Function/4(mode)
  Bus Element In11/1 -> MATLAB Function/5(flag_pos_mode)
  Bus Element In12/1 -> MATLAB Function/6(flag_alt_mode)
  MATLAB Function/1(y) -> Demux1/1
  Demux1/1 -> [des_roll]
  Demux1/2 -> [des_pitch]
  Demux1/3 -> [des_yr]
  Demux1/4 -> Bus Element Out13/1
  Data Type Conversion13/1 -> Bus Element Out15/1
  Data Type Conversion9/1 -> MATLAB Function1/3(in_yawrate)
  Compare To Constant3/1 -> MATLAB Function1/4(flag)
  BusElementIn18/1 -> Data Type Conversion12/1
  MATLAB Function1/1(out_roll) -> Data Type Conversion14/1
  Data Type Conversion10/1 -> MATLAB Function1/6(peak_angle_deg)
  Data Type Conversion2/1 -> MATLAB Function1/1(in_roll)
  PX4 Timestamp/1 -> Data Type Conversion/1
  [des_pitch] -> Data Type Conversion8/1
  MATLAB Function1/3(out_yawrate) -> Data Type Conversion15/1
  BusElementIn16/1 -> Compare To Constant3/1
  Data Type Conversion12/1 -> MATLAB Function1/7(doublet_dt)
  BusElementIn19/1 -> MATLAB Function1/8(doublet_axis)
  [des_yr] -> Data Type Conversion9/1
  Data Type Conversion15/1 -> Bus Element Out16/1
  BusElementIn17/1 -> Data Type Conversion10/1
  Data Type Conversion/1 -> MATLAB Function1/5(time_usec)
  Data Type Conversion8/1 -> MATLAB Function1/2(in_pitch)
  MATLAB Function1/2(out_pitch) -> Data Type Conversion13/1
  [des_roll] -> Data Type Conversion2/1
  Data Type Conversion14/1 -> Bus Element Out14/1
  Demux2/2 -> Bus Element Out10/1
  Demux2/1 -> Bus Element Out17/1
  BusElementIn6/1 -> Subsystem Reference/3
  BusElementIn8/1 -> Subsystem Reference/4
  BusElementIn9/1 -> Subsystem Reference/5
  BusElementIn20/1 -> Subsystem Reference/6
  [reset] -> Subsystem Reference/7
  Bus Element In1/1 -> Subsystem Reference/2
  [ALT_des_vz] -> Subsystem Reference/1
  Subsystem Reference/1 -> MATLAB Function2/1(a_z)  "a_z cmd"
  MATLAB Function2/1(des_throttle) -> [ALT_des_thr], Bus Element Out/1
  BusElementIn10/1 -> MATLAB Function2/2(thr_hover)
  BusElementIn21/1 -> Product/2
  Gain7/1 -> [ALT_des_vz], Bus Element Out5/1
  BusElementIn22/1 -> Product1/2
  BusElementIn23/1 -> Product2/2
  [POS_des_vx] -> Compare To Constant6/1
  AND2/1 -> [POS_Y_reset]
  Bus Element In13/1 -> AND2/1
  BusElementIn24/1 -> Compare To Constant4/1
  Compare To Constant4/1 -> AND2/2
  [POS_des_vy] -> Compare To Constant5/1
  Compare To Constant5/1 -> AND2/3
  Compare To Constant6/1 -> AND1/3
  BusElementIn26/1 -> PID_Altitude1/3
  XOR/1 -> PID_Altitude1/4
  [POS_X_reset] -> XOR/1
  [POS_Y_reset] -> XOR/2
  MATLAB Function3/1(vx_i) -> Bus Element Out7/1, [POS_des_vx]
  MATLAB Function3/2(vy_i) -> Bus Element Out6/1, [POS_des_vy]
  Bus Element In3/1 -> MATLAB Function3/3(heading)
  Gain8/1 -> MATLAB Function3/1(vy_b)
  Gain9/1 -> MATLAB Function3/2(vx_b)
  Discrete PID Controller/1 -> Demux2/1, Sum7/1
  Bus Element In14/1 -> Discrete-Time Integrator/3
  Bus Element In4/1 -> Discrete-Time Integrator1/3
  Discrete-Time Integrator1/1 -> [POS_RC_des_Y]  "des_y"
  Sum4/1 -> Discrete PID Controller/1
  BusElementIn13/1 -> Discrete PID Controller/2
  Mux/1 -> Sum4/1
  [POS_des_Y] -> Mux/2
  [POS_des_X] -> Mux/1
  Mux1/1 -> Sum4/2
  Bus Element In6/1 -> Mux1/1
  Bus Element In7/1 -> Mux1/2
  Sum7/1 -> PID_Altitude1/1
  Bus Element In10/1 -> MATLAB Function4/2(heading)
  MATLAB Function4/1(des_theta) -> [POS_des_pitch], Bus Element Out11/1
  MATLAB Function4/2(des_phi) -> Bus Element Out12/1, [POS_des_roll]
  Bus Element In15/1 -> Mux6/1
  Bus Element In16/1 -> Mux6/2
  Data Type Conversion19/1 -> WPManager/3(L)
  Compare To Constant/1 -> WPManager/4(flag)
  BusElementIn25/1 -> Compare To Constant/1, Switch/2
  WPManager/1(Current_WP) -> Data Type Conversion18/1
  [POS_RC_des_Y] -> Mux7/2
  [POS_RC_des_X] -> Mux7/1
  Mux7/1 -> Switch/3
  Switch/1 -> Demux/1
  Demux/1 -> Bus Element Out8/1, [POS_des_X]
  Demux/2 -> [POS_des_Y], Bus Element Out9/1
  Mux6/1 -> Data Type Conversion16/1
  Bus Element In17/1 -> Data Type Conversion17/1
  Data Type Conversion18/1 -> Switch/1
  Data Type Conversion16/1 -> WPManager/1(X)
  Data Type Conversion17/1 -> WPManager/2(heading)
  BusElementIn28/1 -> Compare To Constant7/1
  BusElementIn29/1 -> Compare To Constant8/1
  Compare To Constant7/1 -> AND1/4
  Compare To Constant8/1 -> AND2/4
  BusElementIn30/1 -> Gain10/1, Discrete PID Controller/3
  Gain10/1 -> Discrete PID Controller/4
  Discrete Varying Lowpass1/1 -> Discrete Derivative1/1
  BusElementIn27/1 -> Product3/1
  Product3/1 -> Sum5/2
  Discrete Derivative1/1 -> Product3/2
  BusElementIn31/1 -> Discrete Varying Lowpass1/2
  PID_Altitude1/1 -> Sum5/1  "az_cmd"
  Sum5/1 -> MATLAB Function4/1(a_cmd)
  BusElementIn32/1 -> Data Type Conversion19/1
